simulink model "Lava_Lamp_Proportional_Control"  (R2016a)
settings: Solver=ode45  StartTime=0.0  StopTime=100000  MaxStep=0.05  RelTol=1e-3
values from neighbouring files (symbols this model uses):
  C1 = 1 / C_HEAT    (= 0.0013206550449)    [ControlDesignAndAnalysis.m]    (also in Lava_Lamp_System_Model.m)
  C2 = 1 / (R123 * C_HEAT)    (= 0.00138569660598)    [ControlDesignAndAnalysis.m]    (also in Lava_Lamp_System_Model.m)
  C3 = 1 / (R1 * C_LAVA)    (= 3.46327878577e-05)    [ControlDesignAndAnalysis.m]    (also in Lava_Lamp_System_Model.m)
  C4 = 1 / (R156 * C_LAVA)    (= 3.89625411326e-05)    [ControlDesignAndAnalysis.m]    (also in Lava_Lamp_System_Model.m)
  C5 = 1/ (R1 * C_HEAT)    (= 0.00137168160044)    [ControlDesignAndAnalysis.m]    (also in Lava_Lamp_System_Model.m)
  K = 10    [Lava_Lamp_System_Model.m]
settings Model: Creator=ddrma  LastModifiedBy=ddrma

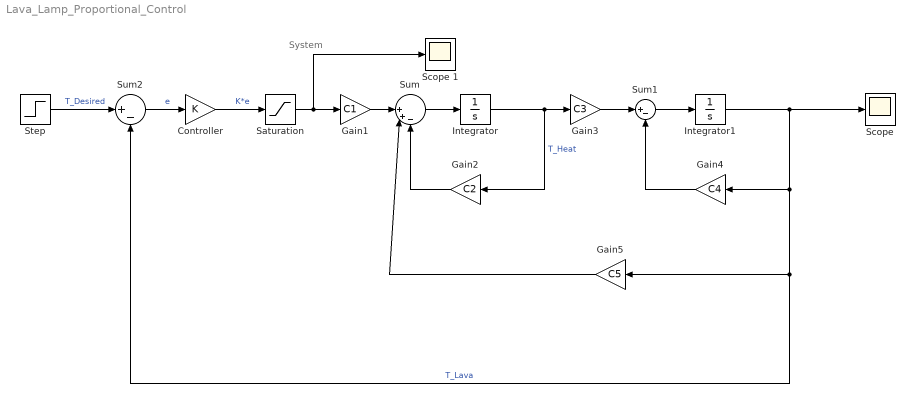
== system Lava_Lamp_Proportional_Control ==
  note: System
  Controller : Gain  Gain=K
  Gain1 : Gain  Gain=C1
  Gain2 : Gain  Gain=C2
  Gain3 : Gain  Gain=C3
  Gain4 : Gain  Gain=C4
  Gain5 : Gain  Gain=C5
  Integrator : Integrator
  Integrator1 : Integrator
  Saturation : Saturate  UpperLimit=64  LowerLimit=0
  "Scope " : Scope
  Scope 1 : Scope
  Step : Step  Time=0  After=40  SampleTime=0
  Sum : Sum  Inputs=||++-
  Sum1 : Sum  Inputs=|+-
  Sum2 : Sum  Inputs=|+-
  wires:
  Sum/1 -> Integrator/1
  Integrator/1 -> Gain3/1, Gain2/1  "T_Heat"
  Gain3/1 -> Sum1/1
  Sum1/1 -> Integrator1/1
  Gain4/1 -> Sum1/2
  Integrator1/1 -> "Scope "/1, Sum2/2, Gain5/1, Gain4/1  "T_Lava"
  Gain2/1 -> Sum/3
  Gain5/1 -> Sum/2
  Gain1/1 -> Sum/1
  Sum2/1 -> Controller/1  "e"
  Saturation/1 -> Scope 1/1, Gain1/1
  Controller/1 -> Saturation/1  "K*e"
  Step/1 -> Sum2/1  "T_Desired"
